simulink subsystem "EVTOL_6DOF_Controller"  (R2025b)
settings: Solver=VariableStepAuto  StartTime=0.0  StopTime=10.0  RelTol=1e-3
undefined symbols (not defined in the file): controller_sample_time, DiscIntNeverNeededParam, gains, MixMatrix, sat
settings Model: Creator=ryanc  LastModifiedBy=ryanc

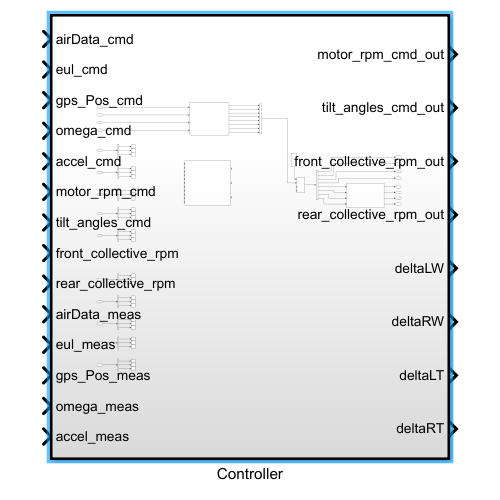
[thumbnail: Simulink's stored preview of the top-level diagram]
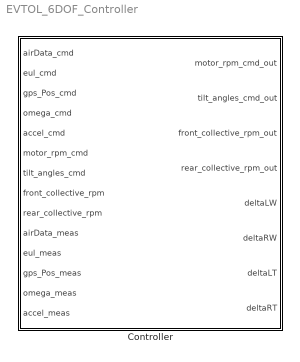
== system EVTOL_6DOF_Controller ==
  Controller : Subsystem  TreatAsAtomicUnit=on  SystemSampleTime=controller_sample_time

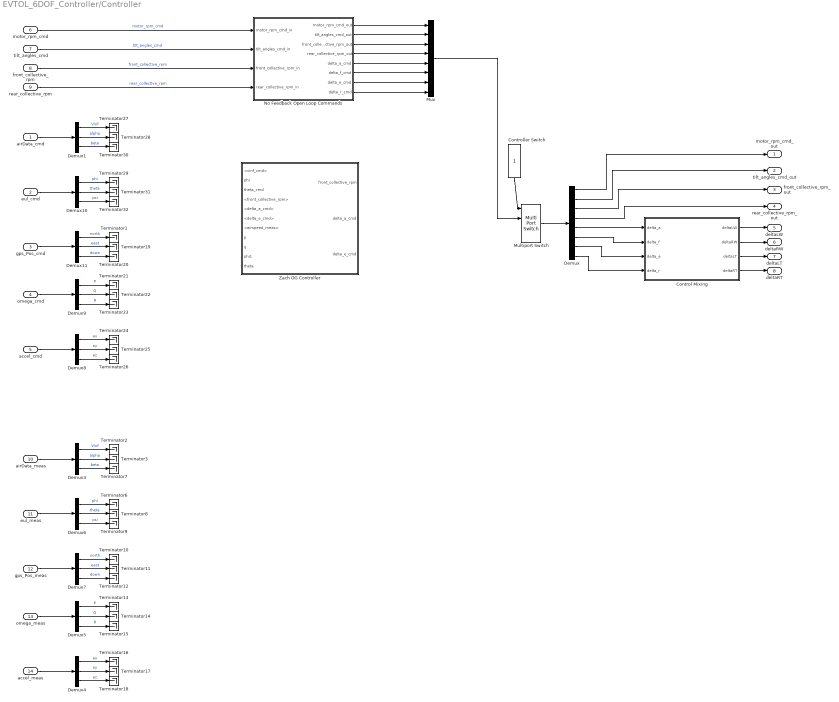
== system EVTOL_6DOF_Controller/Controller ==
  airData_cmd : Inport
  eul_cmd : Inport  Port=2
  gps_Pos_cmd : Inport  Port=3
  omega_cmd : Inport  Port=4
  accel_cmd : Inport  Port=5
  motor_rpm_cmd : Inport  Port=6
  tilt_angles_cmd : Inport  Port=7
  front_collective_rpm : Inport  Port=8
  rear_collective_rpm : Inport  Port=9
  airData_meas : Inport  Port=10
  eul_meas : Inport  Port=11
  gps_Pos_meas : Inport  Port=12
  omega_meas : Inport  Port=13
  accel_meas : Inport  Port=14
  Control Mixing : Subsystem
  Controller Switch : Constant
  Demux : Demux  Outputs=8
  Demux{1,3..11} (10 alike) : Demux  Outputs=3
  Multiport Switch : MultiPortSwitch  SaturateOnIntegerOverflow=off  InputSameDT=off
  Mux : Mux  Inputs=8
  No Feedback Open Loop Commands : Subsystem
  Terminator{1..3,6..32} (30 alike) : Terminator
  Zach OG Controller : Subsystem
  motor_rpm_cmd_out : Outport
  tilt_angles_cmd_out : Outport  Port=2
  front_collective_rpm_out : Outport  Port=3
  rear_collective_rpm_out : Outport  Port=4
  deltaLW : Outport  Port=5
  deltaRW : Outport  Port=6
  deltaLT : Outport  Port=7
  deltaRT : Outport  Port=8
  wires:
  airData_meas/1 -> Demux3/1
  eul_meas/1 -> Demux6/1
  gps_Pos_meas/1 -> Demux7/1
  omega_meas/1 -> Demux5/1
  accel_meas/1 -> Demux4/1
  Demux3/1 -> Terminator2/1  "Vinf"
  Demux3/2 -> Terminator3/1  "alpha"
  Demux3/3 -> Terminator7/1  "beta"
  Demux6/3 -> Terminator9/1  "psi"
  Demux6/1 -> Terminator6/1  "phi"
  Demux6/2 -> Terminator8/1  "theta"
  Demux7/3 -> Terminator12/1  "down"
  Demux7/1 -> Terminator10/1  "north"
  Demux7/2 -> Terminator11/1  "east"
  Demux5/3 -> Terminator15/1  "R"
  Demux5/1 -> Terminator13/1  "P"
  Demux5/2 -> Terminator14/1  "Q"
  Demux4/3 -> Terminator18/1  "az"
  Demux4/1 -> Terminator16/1  "ax"
  Demux4/2 -> Terminator17/1  "ay"
  Demux10/1 -> Terminator29/1  "phi"
  Demux10/3 -> Terminator32/1  "psi"
  Demux1/3 -> Terminator30/1  "beta"
  gps_Pos_cmd/1 -> Demux11/1
  Demux1/1 -> Terminator27/1  "Vinf"
  eul_cmd/1 -> Demux10/1
  omega_cmd/1 -> Demux9/1
  accel_cmd/1 -> Demux8/1
  Demux11/3 -> Terminator20/1  "down"
  Demux11/2 -> Terminator19/1  "east"
  Demux1/2 -> Terminator28/1  "alpha"
  Demux10/2 -> Terminator31/1  "theta"
  Demux9/3 -> Terminator23/1  "R"
  Demux9/1 -> Terminator21/1  "P"
  Demux8/1 -> Terminator24/1  "ax"
  Demux11/1 -> Terminator1/1  "north"
  Demux8/2 -> Terminator25/1  "ay"
  Demux8/3 -> Terminator26/1  "az"
  airData_cmd/1 -> Demux1/1
  Demux9/2 -> Terminator22/1  "Q"
  motor_rpm_cmd/1 -> No Feedback Open Loop Commands/1(motor_rpm_cmd_in)  "motor_rpm_cmd"
  tilt_angles_cmd/1 -> No Feedback Open Loop Commands/2(tilt_angles_cmd_in)  "tilt_angles_cmd"
  rear_collective_rpm/1 -> No Feedback Open Loop Commands/4(rear_collective_rpm_in)  "rear_collective_rpm"
  front_collective_rpm/1 -> No Feedback Open Loop Commands/3(front_collective_rpm_in)  "front_collective_rpm"
  Control Mixing/1(deltaLW) -> deltaLW/1
  Control Mixing/2(deltaRW) -> deltaRW/1
  Control Mixing/3(deltaLT) -> deltaLT/1
  Control Mixing/4(deltaRT) -> deltaRT/1
  Controller Switch/1 -> Multiport Switch/1
  No Feedback Open Loop Commands/6(delta_f_cmd) -> Mux/6
  No Feedback Open Loop Commands/8(delta_r_cmd) -> Mux/8
  No Feedback Open Loop Commands/7(delta_e_cmd) -> Mux/7
  Mux/1 -> Multiport Switch/2
  No Feedback Open Loop Commands/5(delta_a_cmd) -> Mux/5
  No Feedback Open Loop Commands/4(rear_collective_rpm_out) -> Mux/4
  No Feedback Open Loop Commands/3(front_collective_rpm_out) -> Mux/3
  No Feedback Open Loop Commands/2(tilt_angles_cmd_out) -> Mux/2
  No Feedback Open Loop Commands/1(motor_rpm_cmd_out) -> Mux/1
  Multiport Switch/1 -> Demux/1
  Demux/8 -> Control Mixing/4(delta_r)
  Demux/7 -> Control Mixing/3(delta_e)
  Demux/6 -> Control Mixing/2(delta_f)
  Demux/5 -> Control Mixing/1(delta_a)
  Demux/4 -> rear_collective_rpm_out/1
  Demux/3 -> front_collective_rpm_out/1
  Demux/2 -> tilt_angles_cmd_out/1
  Demux/1 -> motor_rpm_cmd_out/1

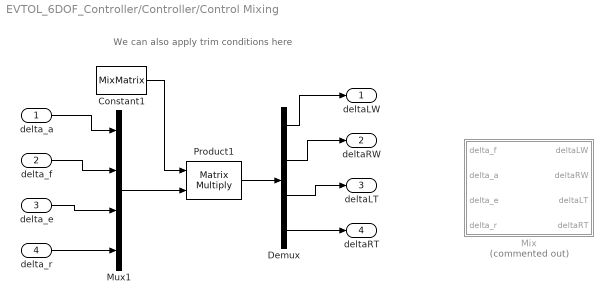
== system EVTOL_6DOF_Controller/Controller/Control Mixing ==
  note: We can also apply trim conditions here
  delta_a : Inport
  delta_f : Inport  Port=2
  delta_e : Inport  Port=3
  delta_r : Inport  Port=4
  Constant1 : Constant  Value=MixMatrix
  Demux : Demux
  Mix : MATLAB Function  Commented=on  TreatAsAtomicUnit=on
  Mux1 : Mux
  Product1 : Product  Multiplication=Matrix(*)
  deltaLW : Outport
  deltaRW : Outport  Port=2
  deltaLT : Outport  Port=3
  deltaRT : Outport  Port=4
  wires:
  delta_a/1 -> Mux1/1
  Demux/1 -> deltaLW/1
  delta_f/1 -> Mux1/2
  Mux1/1 -> Product1/2
  delta_e/1 -> Mux1/3
  Constant1/1 -> Product1/1
  delta_r/1 -> Mux1/4
  Demux/2 -> deltaRW/1
  Product1/1 -> Demux/1
  Demux/3 -> deltaLT/1
  Demux/4 -> deltaRT/1

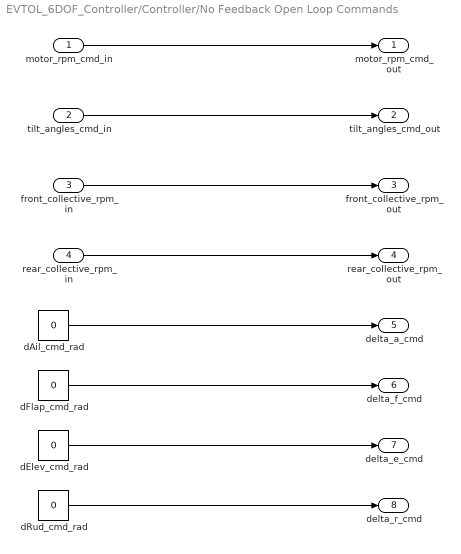
== system EVTOL_6DOF_Controller/Controller/No Feedback Open Loop Commands ==
  motor_rpm_cmd_in : Inport
  tilt_angles_cmd_in : Inport  Port=2
  front_collective_rpm_in : Inport  Port=3
  rear_collective_rpm_in : Inport  Port=4
  dAil_cmd_rad : Constant  Value=0
  dElev_cmd_rad : Constant  Value=0
  dFlap_cmd_rad : Constant  Value=0
  dRud_cmd_rad : Constant  Value=0
  motor_rpm_cmd_out : Outport
  tilt_angles_cmd_out : Outport  Port=2
  front_collective_rpm_out : Outport  Port=3
  rear_collective_rpm_out : Outport  Port=4
  delta_a_cmd : Outport  Port=5  VectorParamsAs1DForOutWhenUnconnected=off
  delta_f_cmd : Outport  Port=6  VectorParamsAs1DForOutWhenUnconnected=off
  delta_e_cmd : Outport  Port=7  VectorParamsAs1DForOutWhenUnconnected=off
  delta_r_cmd : Outport  Port=8  VectorParamsAs1DForOutWhenUnconnected=off
  wires:
  dElev_cmd_rad/1 -> delta_e_cmd/1
  dAil_cmd_rad/1 -> delta_a_cmd/1
  front_collective_rpm_in/1 -> front_collective_rpm_out/1
  rear_collective_rpm_in/1 -> rear_collective_rpm_out/1
  tilt_angles_cmd_in/1 -> tilt_angles_cmd_out/1
  dFlap_cmd_rad/1 -> delta_f_cmd/1
  motor_rpm_cmd_in/1 -> motor_rpm_cmd_out/1
  dRud_cmd_rad/1 -> delta_r_cmd/1

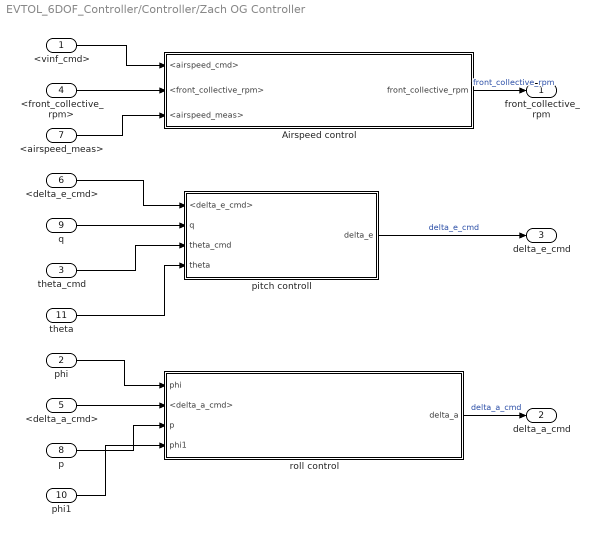
== system EVTOL_6DOF_Controller/Controller/Zach OG Controller ==
  <vinf_cmd> : Inport
  phi : Inport  Port=2
  theta_cmd : Inport  Port=3
  <front_collective_rpm> : Inport  Port=4
  <delta_a_cmd> : Inport  Port=5
  <delta_e_cmd> : Inport  Port=6
  <airspeed_meas> : Inport  Port=7
  p : Inport  Port=8
  q : Inport  Port=9
  phi1 : Inport  Port=10
  theta : Inport  Port=11
  Airspeed control : Subsystem
  pitch controll : Subsystem
  roll control : Subsystem
  front_collective_rpm : Outport
  delta_a_cmd : Outport  Port=2
  delta_e_cmd : Outport  Port=3
  wires:
  <vinf_cmd>/1 -> Airspeed control/1(<airspeed_cmd>)
  <front_collective_rpm>/1 -> Airspeed control/2(<front_collective_rpm>)
  theta/1 -> pitch controll/4(theta)
  <airspeed_meas>/1 -> Airspeed control/3(<airspeed_meas>)
  <delta_e_cmd>/1 -> pitch controll/1(<delta_e_cmd>)
  q/1 -> pitch controll/2(q)
  theta_cmd/1 -> pitch controll/3(theta_cmd)
  phi/1 -> roll control/1(phi)
  <delta_a_cmd>/1 -> roll control/2(<delta_a_cmd>)
  p/1 -> roll control/3(p)
  phi1/1 -> roll control/4(phi1)
  Airspeed control/1(front_collective_rpm) -> front_collective_rpm/1  "front_collective_rpm"
  pitch controll/1(delta_e) -> delta_e_cmd/1  "delta_e_cmd"
  roll control/1(delta_a) -> delta_a_cmd/1  "delta_a_cmd"

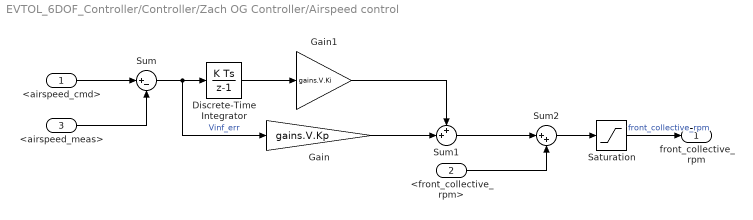
== system EVTOL_6DOF_Controller/Controller/Zach OG Controller/Airspeed control ==
  <airspeed_cmd> : Inport
  <front_collective_rpm> : Inport  Port=2
  <airspeed_meas> : Inport  Port=3
  Discrete-Time Integrator : DiscreteIntegrator  SampleTime=controller_sample_time  LimitOutput=on  UpperSaturationLimit=5000  LowerSaturationLimit=-5000  ICPrevOutput=DiscIntNeverNeededParam  ICPrevScaledInput=DiscIntNeverNeededParam
  Gain : Gain  Gain=gains.V.Kp
  Gain1 : Gain  Gain=gains.V.Ki
  Saturation : Saturate  UpperLimit=sat.frontcollective.high  LowerLimit=sat.frontcollective.low
  Sum : Sum  Inputs=|+-
  Sum1 : Sum  Inputs=++|
  Sum2 : Sum  Inputs=|++
  front_collective_rpm : Outport
  wires:
  <front_collective_rpm>/1 -> Sum2/2
  <airspeed_meas>/1 -> Sum/2
  <airspeed_cmd>/1 -> Sum/1
  Saturation/1 -> front_collective_rpm/1  "front_collective_rpm"
  Sum1/1 -> Sum2/1
  Gain/1 -> Sum1/2
  Gain1/1 -> Sum1/1
  Discrete-Time Integrator/1 -> Gain1/1
  Sum2/1 -> Saturation/1
  Sum/1 -> Gain/1, Discrete-Time Integrator/1  "Vinf_err"

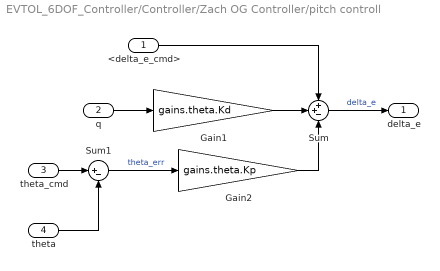
== system EVTOL_6DOF_Controller/Controller/Zach OG Controller/pitch controll ==
  <delta_e_cmd> : Inport
  q : Inport  Port=2
  theta_cmd : Inport  Port=3
  theta : Inport  Port=4
  Gain1 : Gain  Gain=gains.theta.Kd
  Gain2 : Gain  Gain=gains.theta.Kp
  Sum : Sum  Inputs=++-
  Sum1 : Sum  Inputs=|+-
  delta_e : Outport
  wires:
  q/1 -> Gain1/1
  <delta_e_cmd>/1 -> Sum/1
  Sum/1 -> delta_e/1  "delta_e"
  Gain1/1 -> Sum/2
  Gain2/1 -> Sum/3
  theta/1 -> Sum1/2
  theta_cmd/1 -> Sum1/1
  Sum1/1 -> Gain2/1  "theta_err"

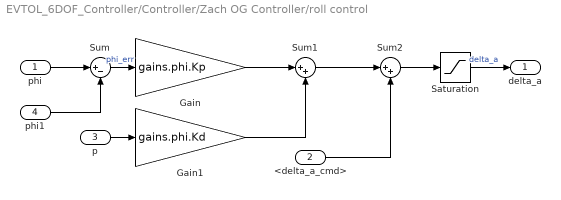
== system EVTOL_6DOF_Controller/Controller/Zach OG Controller/roll control ==
  phi : Inport
  <delta_a_cmd> : Inport  Port=2
  p : Inport  Port=3
  phi1 : Inport  Port=4
  Gain : Gain  Gain=gains.phi.Kp
  Gain1 : Gain  Gain=gains.phi.Kd
  Saturation : Saturate  UpperLimit=sat.delta_a.high  LowerLimit=sat.delta_a.low
  Sum : Sum  Inputs=|+-
  Sum1 : Sum  Inputs=|++
  Sum2 : Sum  Inputs=|++
  delta_a : Outport
  wires:
  <delta_a_cmd>/1 -> Sum2/2
  p/1 -> Gain1/1
  phi/1 -> Sum/1
  Gain1/1 -> Sum1/2
  Gain/1 -> Sum1/1
  Sum/1 -> Gain/1  "phi_err"
  phi1/1 -> Sum/2
  Sum1/1 -> Sum2/1
  Sum2/1 -> Saturation/1
  Saturation/1 -> delta_a/1  "delta_a"

== matlab function EVTOL_6DOF_Controller/Controller/Control Mixing/Mix ==
  data: delta_f input; deltaLW output; delta_a input; delta_e input; delta_r input; deltaRW output; deltaLT output; deltaRT output
function [deltaLW, deltaRW, deltaLT, deltaRT] = fcn(delta_f, delta_a, delta_e, delta_r)
%#codegen
deltaLW = delta_f + delta_a;
deltaRW = delta_f - delta_a;
deltaLT = delta_e - delta_r;
deltaRT = delta_e + delta_r;
end
